simulink model "flightplan2"  (R2021b)
settings: Solver=VariableStepAuto  StartTime=0.0  StopTime=10.0  RelTol=1e-3
settings Model: Creator=verti  LastModifiedBy=verti

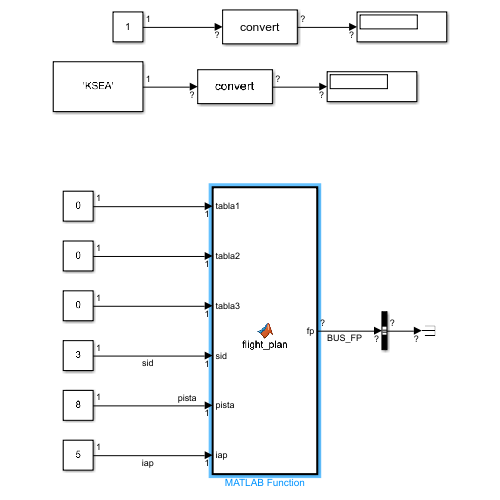
[thumbnail: Simulink's stored preview of the top-level diagram]
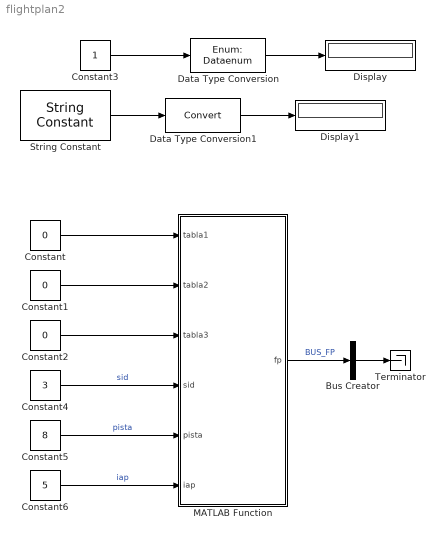
== system flightplan2 ==
  Bus Creator : BusCreator  Inputs=1
  Constant : Constant  Value=0  OutDataTypeStr=Bus: BUS_SID
  Constant1 : Constant  Value=0  OutDataTypeStr=Bus: BUS_WP
  Constant2 : Constant  Value=0  OutDataTypeStr=Bus: BUS_IAP
  Constant3 : Constant  OutDataTypeStr=int32
  Constant4 : Constant  Value=3
  Constant5 : Constant  Value=8
  Constant6 : Constant  Value=5
  Data Type Conversion : DataTypeConversion  OutDataTypeStr=Enum: Dataenum
  Data Type Conversion1 : DataTypeConversion
  Display : Display
  Display1 : Display
  MATLAB Function : MATLAB Function  TreatAsAtomicUnit=on
  String Constant : StringConstant  String='KSEA'
  Terminator : Terminator
  wires:
  Constant3/1 -> Data Type Conversion/1
  Data Type Conversion/1 -> Display/1
  String Constant/1 -> Data Type Conversion1/1
  Data Type Conversion1/1 -> Display1/1
  Constant/1 -> MATLAB Function/1(tabla1)
  Constant1/1 -> MATLAB Function/2(tabla2)
  Constant5/1 -> MATLAB Function/5(pista)  "pista"
  Constant4/1 -> MATLAB Function/4(sid)  "sid"
  Constant2/1 -> MATLAB Function/3(tabla3)
  MATLAB Function/1(fp) -> Bus Creator/1  "BUS_FP"
  Constant6/1 -> MATLAB Function/6(iap)  "iap"
  Bus Creator/1 -> Terminator/1

== matlab function flightplan2/MATLAB Function ==
  data: tabla1 input Bus: BUS_SID; tabla2 input Bus: BUS_WP; tabla3 input Bus: BUS_IAP; sid input; fp output Bus: BUS_FP; pista input; iap input
function fp  = flight_plan(tabla1,tabla2,tabla3,sid,pista,iap)

% Hay que proporcionarle 3 cadenas de carácteres SID,Pista de SID y el IAP.
% EJEMPLO: fp = flight_plan(tabla1,tabla2,tabla3,3,8,5)

%% Antes de usar
%{
tabla1 = readtable('SIDs.xlsx');
tabla2 = readtable('WPs.xlsx');
tabla3 = readtable('IAPs.xlsx');
tabla1=table2struct(tabla1);
tabla2=table2struct(tabla2);
tabla3=table2struct(tabla3);
%}
%% Creación plan de vuelo (en tabla)

t111 = tabla1([tabla1.SID] == sid);
t11 = t111([t111.Runway] == pista);
%t1 = rmfield(rmfield(rmfield(t11,'Airport'),'SID'),'Runway');
t33 = tabla3([tabla3.SID] == iap); %%%%%%%%%%%%%%%%%IAP
%t3 = rmfield(rmfield(rmfield(t33,'Airport'),'IAP'),'Runway');
fp=[t11;t33];

%% Cálculo de distancias entre waypoints

for i=2:length(fp)
    fp(i).Leg_distance=60*distance('gc',fp(i).Latitude,fp(i).Longitude,fp(i-1).Latitude,fp(i-1).Longitude);
end


end
